simulink model "PID2"  (R2020b)
settings: Solver=FixedStepAuto  StartTime=0.0  StopTime=5  FixedStep=0.001  RelTol=1e-3
libraries: simulink_extras x2, shared3dof x1, SignalEditorBlockLib x1, simulink x1
settings Model: NumberOfSteps=25  OrderedModelArguments=off  Creator=Daniel Alstrup  LastModifiedBy=Daniel Alstrup

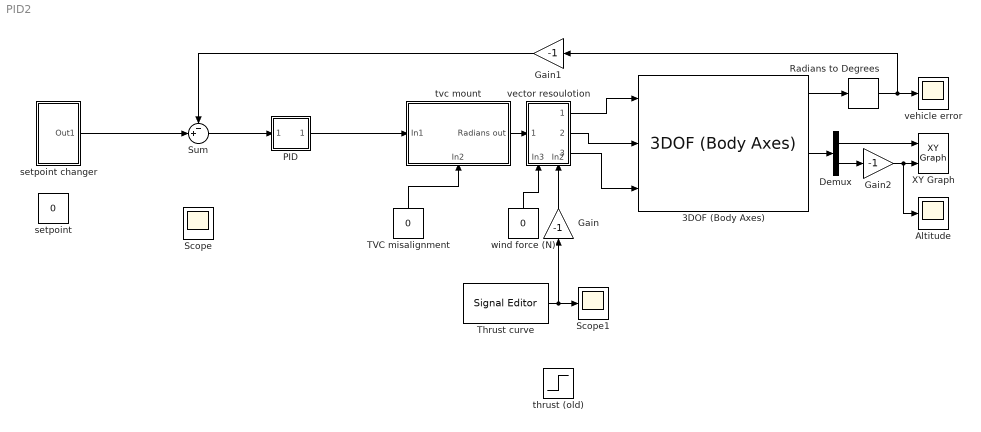
== system PID2 ==
  3DOF (Body Axes) : shared3dof/3DOF (Body Axes)  units=Metric (MKS)  mtype=Fixed  v_ini=0  theta_ini=0  alpha_ini=0  pos_ini=[0 0]  q_ini=0  mass=0.834  mass_e=0.5  mass_f=3.0  Iyy=0.1366  Iyy_e=0.5  Iyy_f=3.0  g_in=Internal  g=9.81  vre_flag=on  abi_flag=off  aMode=0  vel_statename=''  theta_statename=''  pos_statename=''  q_statename=''  mass_statename=''
      settings: SourceProductBaseCode=AE,PW,MT,UV,VE,VP
  Altitude : Scope
  Demux : Demux  Outputs=2
  Gain : Gain  Gain=-1
  Gain1 : Gain  Gain=-1
  Gain2 : Gain  Gain=-1
  PID : Subsystem
  Radians to Degrees : simulink_extras/Transformations/Radians to Degrees
  Scope : Scope
  Scope1 : Scope
  Sum : Sum  Inputs=-+|
  TVC misalignment : Constant  Value=0
  Thrust curve : SignalEditorBlockLib/Signal Editor  FileName=untitled.mat  ActiveScenario=Scenario  ActiveSignal=F-15 thrust curve  IsBus=off  OutputBusObjectStr=Bus: BusObject  SampleTime=0  ZeroCross=off  OutputAfterFinalValue=Setting to zero  Unit=inherit  PreserveSignalName=on
  XY Graph : simulink/Sinks/XY Graph  xmin=-50  xmax=50  ymin=-1  ymax=200  st=-1
  setpoint : Constant  Value=0
  setpoint changer : Subsystem
  "thrust (old) " : Step  Time=5  Before=-15  After=0  SampleTime=0
  tvc mount : Subsystem
      settings: PortSchema="{\"entries\":[{\"content\":{\"sides\":[{\"content\":{\"connectorIds\":[\"In1\"]},\"type\":\"ConnectorPlacement.EquallySpacedRectSide\",\"uuid\":\"7db720e9-f193-4667-a462-54aba387b780\"},{\"content\":{\"connectorIds\":[\"Out1\"],\"side\":\"RIGHT\"},\"type\":\"ConnectorPlacement.EquallySpacedRectSide\",\"uuid\":\"0b813e1d-285d-4ec7-8b35-0b146b391fcd\"},{\"content\":{\"connectorIds\":[],\"side\":\"TOP\"},\"type\":\"ConnectorPlacement.EquallySpacedRectSide\",\"uuid\":\"87bd1fb0-677d-4d38-906e-fbf3f7328a0b\"},{\"content\":{\"connectorIds\":[\"In2\"],\"side\":\"BOTTOM\"},\"type\":\"ConnectorPlacement.EquallySpacedRectSide\",\"uuid\":\"4210e64a-cbef-438e-97fa-a40bfcd5aead\"},{\"content\":{\"connectorIds\":[],\"side\":\"HIDDEN\"},\"type\":\"ConnectorPlacement.EquallySpacedRectSide\",\"uuid\":\"e5f28b75-937b-4906-8744-70272fba026a\"}]},\"type\":\"ConnectorPlacement.EquallySpacedConnector\",\"uuid\":\"6bedd382-364c-4197-a250-851569a75bfe\"}],\"packageUris\":[\"http://schema.mathworks.com/mf0/Connector/R2020b\"],\"version\":\"1.0\"}"
  vector resoulotion : Subsystem
      settings: PortSchema="{\"entries\":[{\"content\":{\"sides\":[{\"content\":{\"connectorIds\":[\"In1\"]},\"type\":\"ConnectorPlacement.EquallySpacedRectSide\",\"uuid\":\"96906159-bd66-4e9d-8d31-c4799863f52b\"},{\"content\":{\"connectorIds\":[\"Out1\",\"Out2\",\"Out3\"],\"side\":\"RIGHT\"},\"type\":\"ConnectorPlacement.EquallySpacedRectSide\",\"uuid\":\"e84a32d2-1cb5-47d4-af10-b137d7c35bba\"},{\"content\":{\"connectorIds\":[],\"side\":\"TOP\"},\"type\":\"ConnectorPlacement.EquallySpacedRectSide\",\"uuid\":\"7099a6d3-5da4-4551-8ca8-9e34e068e228\"},{\"content\":{\"connectorIds\":[\"In2\",\"In3\"],\"side\":\"BOTTOM\"},\"type\":\"ConnectorPlacement.EquallySpacedRectSide\",\"uuid\":\"c923dcc6-b083-4ed3-9ff3-ce9536e74abe\"},{\"content\":{\"connectorIds\":[],\"side\":\"HIDDEN\"},\"type\":\"ConnectorPlacement.EquallySpacedRectSide\",\"uuid\":\"4e828b16-6e7f-4122-84dc-790ac17b6f30\"}]},\"type\":\"ConnectorPlacement.EquallySpacedConnector\",\"uuid\":\"83f65023-5bf0-482e-9d3c-9e5f7b887946\"}],\"packageUris\":[\"http://schema.mathworks.com/mf0/Connector/R2020b\"],\"version\":\"1.0\"}"
  vehicle error : Scope
  wind force (N) : Constant  Value=0
  wires:
  3DOF (Body Axes)/1 -> Radians to Degrees/1
  Radians to Degrees/1 -> Gain1/1, vehicle error/1
  Gain2/1 -> Altitude/1, XY Graph/2
  3DOF (Body Axes)/4 -> Demux/1
  Demux/2 -> Gain2/1
  vector resoulotion/1(Out1) -> 3DOF (Body Axes)/1
  tvc mount/1(Radians out) -> vector resoulotion/1(In1)
  vector resoulotion/3(Out3) -> 3DOF (Body Axes)/3
  Demux/1 -> XY Graph/1
  wind force (N)/1 -> vector resoulotion/2(In3)
  Gain1/1 -> Sum/1
  vector resoulotion/2(Out2) -> 3DOF (Body Axes)/2
  TVC misalignment/1 -> tvc mount/2(In2)
  Gain/1 -> vector resoulotion/3(In2)
  Thrust curve/1 -> Scope1/1, Gain/1
  PID/1(Out1) -> tvc mount/1(In1)
  Sum/1 -> PID/1(In1)
  setpoint changer/1(Out1) -> Sum/2

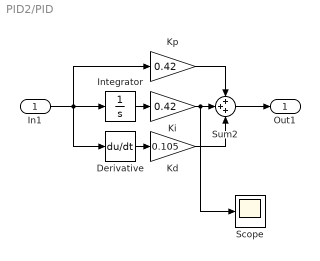
== system PID2/PID ==
  In1 : Inport
  Derivative : Derivative
  Integrator : Integrator  LimitOutput=on  UpperSaturationLimit=27  LowerSaturationLimit=-27
  Kd : Gain  Gain=0.105
  Ki : Gain  Gain=0.42
  Kp : Gain  Gain=0.42
  Scope : Scope
  Sum2 : Sum  Inputs=+++
  Out1 : Outport
  wires:
  Sum2/1 -> Out1/1
  In1/1 -> Integrator/1, Kp/1, Derivative/1
  Kp/1 -> Sum2/1
  Kd/1 -> Sum2/3
  Ki/1 -> Scope/1, Sum2/2
  Derivative/1 -> Kd/1
  Integrator/1 -> Ki/1

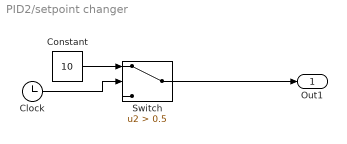
== system PID2/setpoint changer ==
  Clock : Clock
  Constant : Constant  Value=10
  Switch : Switch  Criteria=u2 > Threshold  Threshold=0.5
  Out1 : Outport
  wires:
  Constant/1 -> Switch/1
  Switch/1 -> Out1/1
  Clock/1 -> Switch/2

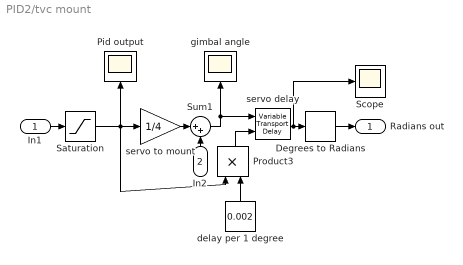
== system PID2/tvc mount ==
  In1 : Inport
  In2 : Inport  Port=2
  Degrees to Radians : simulink_extras/Transformations/Degrees to Radians
  Pid output : Scope
  Product3 : Product
  Saturation : Saturate  UpperLimit=30  LowerLimit=-30
  Scope : Scope
  Sum1 : Sum  Inputs=|++
  delay per 1 degree : Constant  Value=0.002
  gimbal angle : Scope
  servo delay : VariableTransportDelay  MaximumDelay=0.12
  servo to mount : Gain  Gain=1/4
  Radians out : Outport
  wires:
  servo delay/1 -> Scope/1, Degrees to Radians/1
  Product3/1 -> servo delay/2
  servo to mount/1 -> Sum1/1
  Saturation/1 -> Product3/1, Pid output/1, servo to mount/1
  In1/1 -> Saturation/1
  Degrees to Radians/1 -> Radians out/1
  delay per 1 degree/1 -> Product3/2
  Sum1/1 -> gimbal angle/1, servo delay/1
  In2/1 -> Sum1/2

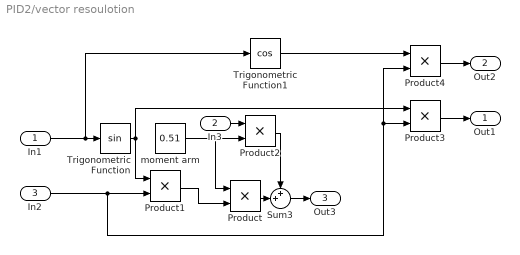
== system PID2/vector resoulotion ==
  In1 : Inport
  In3 : Inport  Port=2
  In2 : Inport  Port=3
  Product{,1..4} (5 alike) : Product
  Sum3 : Sum  Inputs=++|
  Trigonometric Function : Trigonometry
  Trigonometric Function1 : Trigonometry  Operator=cos
  moment arm : Constant  Value=0.51
  Out1 : Outport
  Out2 : Outport  Port=2
  Out3 : Outport  Port=3
  wires:
  In1/1 -> Trigonometric Function1/1, Trigonometric Function/1
  Sum3/1 -> Out3/1
  Product/1 -> Sum3/2
  Trigonometric Function/1 -> Product3/1, Product1/1
  In2/1 -> Product4/2, Product3/2, Product1/2
  moment arm/1 -> Product/1, Product2/2
  Product1/1 -> Product/2
  Product2/1 -> Sum3/1
  Product4/1 -> Out2/1
  Trigonometric Function1/1 -> Product4/1
  Product3/1 -> Out1/1
  In3/1 -> Product2/1
